simulink model "ML"  (R2022a)
settings: Solver=ode2  StartTime=0.0  StopTime=30  FixedStep=0.1  RelTol=1e-3  EnableMultiTasking=on
values from neighbouring files (symbols this model uses):
  Cm = 20    [ML_parameter.m]
  fai = 0.066    [ML_parameter.m]
  g_Ca = 4.4    [ML_parameter.m]
  g_K = 8    [ML_parameter.m]
  g_L = 0.2    [ML_parameter.m]
  V1 = -1    [ML_parameter.m]
  V2 = 15    [ML_parameter.m]
  V3 = 2    [ML_parameter.m]
  V4 = 30    [ML_parameter.m]
  V_Ca = 100    [ML_parameter.m]
  V_K = 70    [ML_parameter.m]
  V_L = 50    [ML_parameter.m]
settings Model: Creator=Administrator  LastModifiedBy=Anoth
settings SolverCC: AlgebraicLoopSolver=TrustRegion
settings DataIOCC: LimitDataPoints=on  SaveFormat=Array  SignalLoggingSaveFormat=ModelDataLogs  ReturnWorkspaceOutputs=off
settings OptimizationCC: ExpressionDepthLimit=2147483647  InitFltsAndDblsToZero=on  LifeSpan=inf
settings DebuggingCC: UnderspecifiedInitializationDetection=Classic  MergeDetectMultiDrivingBlocksExec=none  SolverPrmCheckMsg=warning  FcnCallInpInsideContextMsg=warning  UnconnectedInputMsg=warning  UnconnectedOutputMsg=warning  UnconnectedLineMsg=warning  StateNameClashWarn=warning  SFUnexpectedBacktrackingDiag=warning  SFNoUnconditionalDefaultTransitionDiag=warning  SFExecutionAtInitializationDiag=none  SFMachineParentedDataDiag=warning  ArithmeticOperatorsInVariantConditions=warning
settings HardwareCC: ProdBitPerPointer=32  ProdBitPerSizeT=32  ProdBitPerPtrDiffT=32  ProdLargestAtomicFloat=None  ProdIntDivRoundTo=Undefined  ProdEndianess=Unspecified  ProdWordSize=32  ProdHWDeviceType=32-bit Generic
settings ModelReferenceCC: PropagateSignalLabelsOutOfModel=off
settings CodeAppCC: StateflowObjectComments=on
settings GRTTargetCC: TargetLangStandard=C89/C90 (ANSI)  CombineOutputUpdateFcns=off  GRTInterface=on
settings ConfigComp: CovMetricSettings=dw  CovSaveCumulativeToWorkspaceVar=on  CovSaveSingleToWorkspaceVar=on

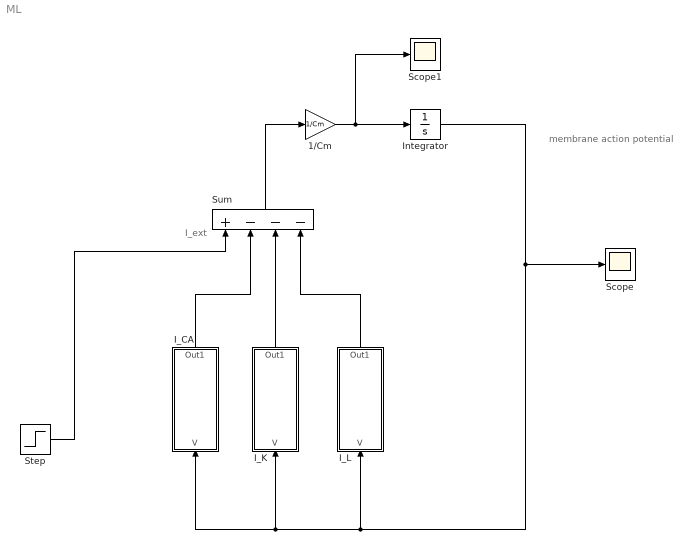
== system ML ==
  note: membrane action potential
  note: I_ext
  1/Cm : Gain  Gain=1/Cm
  "I_CA " : Subsystem
  I_K : Subsystem
  I_L : Subsystem
  Integrator : Integrator  InitialCondition=-10
  Scope : Scope
  Scope1 : Scope
  Step : Step  Time=0  After=100  SampleTime=0
  Sum : Sum  Inputs=+---
  wires:
  Integrator/1 -> I_L/1(V), I_K/1(V), "I_CA "/1(V), Scope/1
  Sum/1 -> 1/Cm/1
  I_L/1(Out1) -> Sum/4
  I_K/1(Out1) -> Sum/3
  "I_CA "/1(Out1) -> Sum/2
  1/Cm/1 -> Scope1/1, Integrator/1
  Step/1 -> Sum/1

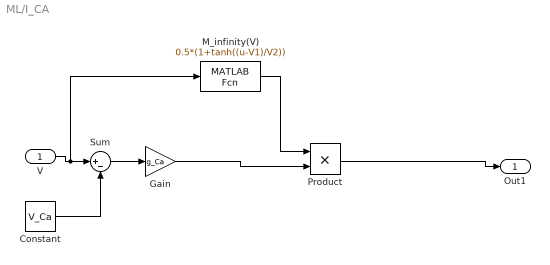
== system ML/I_CA  ==
  V : Inport
  Constant : Constant  Value=V_Ca
  Gain : Gain  Gain=g_Ca
  M_infinity(V) : MATLABFcn  MATLABFcn=0.5*(1+tanh((u-V1)/V2))
  Product : Product  RndMeth=Zero
  Sum : Sum  Inputs=|+-
  Out1 : Outport
  wires:
  V/1 -> Sum/1, M_infinity(V)/1
  Constant/1 -> Sum/2
  Sum/1 -> Gain/1
  Gain/1 -> Product/2
  M_infinity(V)/1 -> Product/1
  Product/1 -> Out1/1

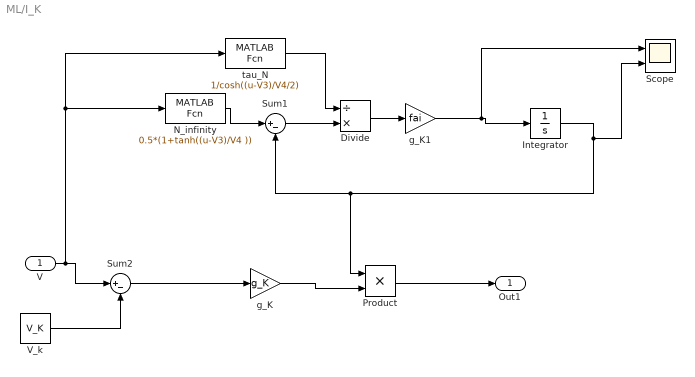
== system ML/I_K ==
  V : Inport
  Divide : Product  Inputs=/*
  Integrator : Integrator
  N_infinity : MATLABFcn  MATLABFcn=0.5*(1+tanh((u-V3)/V4 ))
  Product : Product  RndMeth=Zero
  Scope : Scope  NumInputPorts=2
  Sum1 : Sum  Inputs=|+-
  Sum2 : Sum  Inputs=|+-
  V_k : Constant  Value=V_K
  g_K : Gain  Gain=g_K
  g_K1 : Gain  Gain=fai
  tau_N : MATLABFcn  MATLABFcn=1/cosh((u-V3)/V4/2)
  Out1 : Outport
  wires:
  V/1 -> tau_N/1, N_infinity/1, Sum2/1
  V_k/1 -> Sum2/2
  N_infinity/1 -> Sum1/1
  Integrator/1 -> Scope/2, Sum1/2, Product/1
  tau_N/1 -> Divide/1
  Sum1/1 -> Divide/2
  Divide/1 -> g_K1/1
  g_K1/1 -> Scope/1, Integrator/1
  Sum2/1 -> g_K/1
  g_K/1 -> Product/2
  Product/1 -> Out1/1

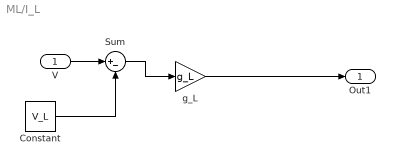
== system ML/I_L ==
  V : Inport
  Constant : Constant  Value=V_L
  Sum : Sum  Inputs=|+-
  g_L : Gain  Gain=g_L
  Out1 : Outport
  wires:
  V/1 -> Sum/1
  Constant/1 -> Sum/2
  Sum/1 -> g_L/1
  g_L/1 -> Out1/1
